simulink model "vectoring2023"  (R2023b)
settings: Solver=FixedStepAuto  StartTime=0.0  StopTime=10  FixedStep=0.001  RelTol=1e-3
undefined symbols (not defined in the file): DiscIntNeverNeededParam
libraries: simulink x4
(part 1 of 2)
settings Model: Creator=manda  LastModifiedBy=manda
settings DebuggingCC: AlgebraicLoopMsg=none  ArtificialAlgebraicLoopMsg=none
settings RTWCC: GPUComputeCapability=5.0

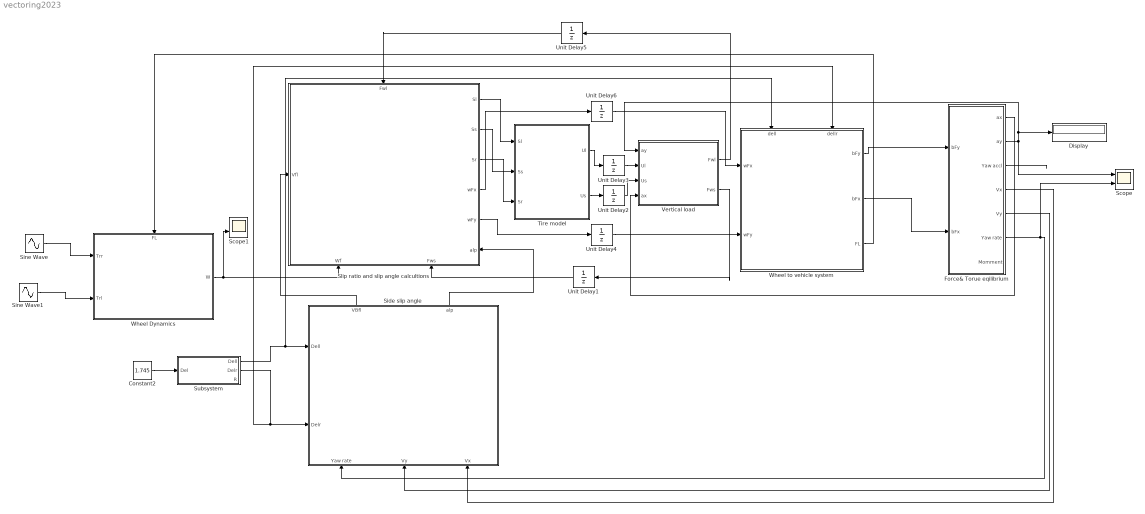
== system vectoring2023 ==
  Constant2 : Constant  Value=1.745
  Display : Display
  Force& Torue eqilibrium : Subsystem
  Scope : Scope  NumInputPorts=2
  Scope1 : Scope  NumInputPorts=2
  Side slip angle : Subsystem
      settings: PortSchema="{\"entries\":[{\"content\":{\"sides\":[{\"content\":{\"connectorIds\":[\"In1\",\"In2\",\"In3\"]},\"type\":\"ConnectorPlacement.EquallySpacedRectSide\",\"uuid\":\"ab28ffba-4240-48bb-9504-9e35b52ca467\"},{\"content\":{\"connectorIds\":[\"Out1\",\"Out2\"],\"side\":\"RIGHT\"},\"type\":\"ConnectorPlacement.EquallySpacedRectSide\",\"uuid\":\"e82fd81c-35f0-42c8-ade2-8771ec67db7c\"},{\"content\":{\"side\":\"TOP\"},\"type\":\"ConnectorPlacement.EquallySpacedRectSide\",\"uuid\":\"b58f2881-2655-4ae0-b45f-be5580c20129\"},{\"content\":{\"connectorIds\":[\"In4\",\"In5\"],\"side\":\"BOTTOM\"},\"type\":\"ConnectorPlacement.EquallySpacedRectSide\",\"uuid\":\"e7768be2-30e0-47b0-bc7d-0a1efc3645f2\"}]},\"type\":\"ConnectorPlacement.EquallySpacedConnector\",\"uuid\":\"813aa404-2cb1-4c8d-a503-6d07b8fe7df3\"}],\"packageUris\":[\"http://schema.mathworks.com/mf0/Connector/R2020b\"],\"version\":\"1.0\"}"
  Sine Wave : Sin  Amplitude=300  SampleTime=0
  Sine Wave1 : Sin  Amplitude=280  Frequency=2  SampleTime=0
  Slip ratio and slip angle calcultions : Subsystem
      settings: PortSchema="{\"entries\":[{\"content\":{\"sides\":[{\"content\":{\"connectorIds\":[\"In1\"]},\"type\":\"ConnectorPlacement.EquallySpacedRectSide\",\"uuid\":\"a7ec119f-fde6-41d0-ac79-405e8e24b01a\"},{\"content\":{\"connectorIds\":[\"Out1\",\"Out2\",\"Out3\",\"Out4\",\"Out5\",\"In5\"],\"side\":\"RIGHT\"},\"type\":\"ConnectorPlacement.EquallySpacedRectSide\",\"uuid\":\"f3b150d3-40b1-4a48-adf8-cf1c21578111\"},{\"content\":{\"connectorIds\":[\"In2\"],\"side\":\"TOP\"},\"type\":\"ConnectorPlacement.EquallySpacedRectSide\",\"uuid\":\"012c84a0-3b90-4200-9e2e-18642f8e7c8c\"},{\"content\":{\"connectorIds\":[\"In3\",\"In4\"],\"side\":\"BOTTOM\"},\"type\":\"ConnectorPlacement.EquallySpacedRectSide\",\"uuid\":\"07872eaa-713c-4fe8-8440-cce3cb3174e0\"}]},\"type\":\"ConnectorPlacement.EquallySpacedConnector\",\"uuid\":\"20f169d6-3b99-4690-9979-164201d75b1c\"}],\"packageUris\":[\"http://schema.mathworks.com/mf0/Connector/R2020b\"],\"version\":\"1.0\"}"
  Subsystem : Subsystem
  Tire model : Subsystem
  Unit Delay{1..6} (6 alike) : UnitDelay  SampleTime=-1  HasFrameUpgradeWarning=on
  "Vertical load " : Subsystem
  Wheel Dynamics : Subsystem
      settings: PortSchema="{\"entries\":[{\"content\":{\"sides\":[{\"content\":{\"connectorIds\":[\"In1\",\"In2\"]},\"type\":\"ConnectorPlacement.EquallySpacedRectSide\",\"uuid\":\"b5deda4c-2c89-449a-b9af-669b3c34e6b4\"},{\"content\":{\"connectorIds\":[\"Out1\"],\"side\":\"RIGHT\"},\"type\":\"ConnectorPlacement.EquallySpacedRectSide\",\"uuid\":\"37e39622-b3a7-494f-b6c8-82365593df34\"},{\"content\":{\"connectorIds\":[\"In3\"],\"side\":\"TOP\"},\"type\":\"ConnectorPlacement.EquallySpacedRectSide\",\"uuid\":\"023e6718-854f-4ad6-a520-bdc192d9d93c\"}]},\"type\":\"ConnectorPlacement.EquallySpacedConnector\",\"uuid\":\"2e43a3da-411d-4540-923d-79338234d95c\"}],\"packageUris\":[\"http://schema.mathworks.com/mf0/Connector/R2020b\"],\"version\":\"1.0\"}"
  Wheel to vehicle system : Subsystem
      settings: PortSchema="{\"entries\":[{\"content\":{\"sides\":[{\"content\":{\"connectorIds\":[\"In1\",\"In2\"]},\"type\":\"ConnectorPlacement.EquallySpacedRectSide\",\"uuid\":\"5c83ab18-6927-4337-9510-166b24334d1c\"},{\"content\":{\"connectorIds\":[\"Out1\",\"Out2\",\"Out3\"],\"side\":\"RIGHT\"},\"type\":\"ConnectorPlacement.EquallySpacedRectSide\",\"uuid\":\"a6e62921-01da-4957-9ce0-76b671842a08\"},{\"content\":{\"connectorIds\":[\"In3\",\"In4\"],\"side\":\"TOP\"},\"type\":\"ConnectorPlacement.EquallySpacedRectSide\",\"uuid\":\"6fd248c4-32bd-4a33-9140-17907c8186f8\"}]},\"type\":\"ConnectorPlacement.EquallySpacedConnector\",\"uuid\":\"96144e17-0eac-422a-892f-fd6e2a88ebc7\"}],\"packageUris\":[\"http://schema.mathworks.com/mf0/Connector/R2020b\"],\"version\":\"1.0\"}"
  wires:
  Slip ratio and slip angle calcultions/3(Sr) -> Tire model/3(Sr)
  "Vertical load "/1(Fwl) -> Unit Delay5/1
  Subsystem/1(Dell) -> Wheel to vehicle system/3(dell), Side slip angle/5(Dell)
  Subsystem/2(Delr) -> Side slip angle/4(Delr), Wheel to vehicle system/4(dellr)
  Constant2/1 -> Subsystem/1(Del)
  Force& Torue eqilibrium/6(Yaw rate) -> Scope/2, Side slip angle/3(Yaw rate)
  Force& Torue eqilibrium/1(ax) -> "Vertical load "/4(ax)
  Force& Torue eqilibrium/2(ay) -> "Vertical load "/1(ay), Display/1, Scope/1
  Side slip angle/1(alp) -> Slip ratio and slip angle calcultions/5(alp)
  Side slip angle/2(VBfl) -> Slip ratio and slip angle calcultions/1(Vfl)
  Slip ratio and slip angle calcultions/1(Sl) -> Tire model/1(Sl)
  Slip ratio and slip angle calcultions/2(Ss) -> Tire model/2(Ss)
  Force& Torue eqilibrium/4(Vx) -> Side slip angle/1(Vx)
  Force& Torue eqilibrium/5(Vy) -> Side slip angle/2(Vy)
  Sine Wave/1 -> Wheel Dynamics/1(Trr)
  Sine Wave1/1 -> Wheel Dynamics/2(Trl)
  Wheel Dynamics/1(W) -> Scope1/2, Slip ratio and slip angle calcultions/3(Wf)
  Tire model/2(Us) -> Unit Delay2/1
  Unit Delay2/1 -> "Vertical load "/3(Us)
  Tire model/1(Ul) -> Unit Delay3/1
  Unit Delay3/1 -> "Vertical load "/2(Ul)
  Unit Delay5/1 -> Slip ratio and slip angle calcultions/2(Fwl)
  Slip ratio and slip angle calcultions/5(wFy) -> Unit Delay4/1
  Slip ratio and slip angle calcultions/4(wFx) -> Unit Delay6/1
  "Vertical load "/2(Fws) -> Unit Delay1/1
  Unit Delay1/1 -> Slip ratio and slip angle calcultions/4(Fws)
  Unit Delay4/1 -> Wheel to vehicle system/2(wFy)
  Unit Delay6/1 -> Wheel to vehicle system/1(wFx)
  Wheel to vehicle system/1(bFy) -> Force& Torue eqilibrium/1(bFy)
  Wheel to vehicle system/2(bFx) -> Force& Torue eqilibrium/2(bFx)
  Force& Torue eqilibrium/3(Yaw accl) -> ?
  Wheel to vehicle system/3(FL) -> Wheel Dynamics/3(FL)

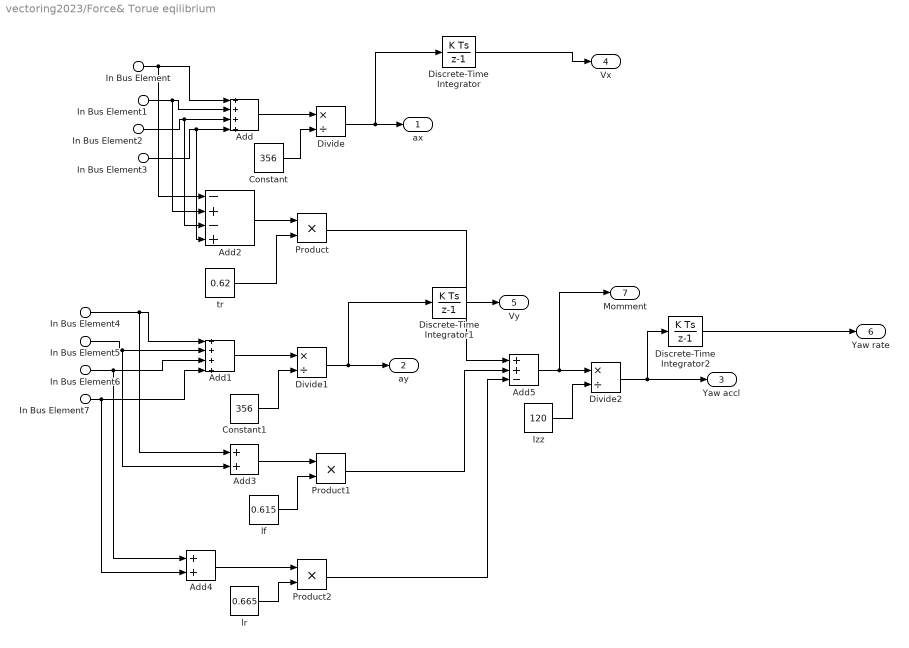
== system vectoring2023/Force& Torue eqilibrium ==
  In Bus Element4 : Inport  PortName=bFy  Element=bFy;fl
  In Bus Element5 : Inport  PortName=bFy  Element=bFy;fr
  In Bus Element6 : Inport  PortName=bFy  Element=Fwy;rl
  In Bus Element7 : Inport  PortName=bFy  Element=Fwy;rr
  In Bus Element : Inport  Port=2  PortName=bFx  Element=bFx;fl
  In Bus Element1 : Inport  Port=2  PortName=bFx  Element=bFx;fr
  In Bus Element2 : Inport  Port=2  PortName=bFx  Element=Fwx;rl
  In Bus Element3 : Inport  Port=2  PortName=bFx  Element=Fwx;rr
  Add : Sum  Inputs=++++
  Add1 : Sum  Inputs=++++
  Add2 : Sum  Inputs=-+-+
  Add3 : Sum
  Add4 : Sum
  Add5 : Sum  Inputs=++-
  Constant : Constant  Value=356
  Constant1 : Constant  Value=356
  Discrete-Time Integrator : DiscreteIntegrator  SampleTime=-1  ICPrevOutput=DiscIntNeverNeededParam  ICPrevScaledInput=DiscIntNeverNeededParam
  Discrete-Time Integrator1 : DiscreteIntegrator  SampleTime=-1  ICPrevOutput=DiscIntNeverNeededParam  ICPrevScaledInput=DiscIntNeverNeededParam
  Discrete-Time Integrator2 : DiscreteIntegrator  SampleTime=-1  ICPrevOutput=DiscIntNeverNeededParam  ICPrevScaledInput=DiscIntNeverNeededParam
  Divide : Product  Inputs=*/
  Divide1 : Product  Inputs=*/
  Divide2 : Product  Inputs=*/
  Izz : Constant  Value=120
  Product : Product
  Product1 : Product
  Product2 : Product
  lf : Constant  Value=0.615
  lr : Constant  Value=0.665
  tr : Constant  Value=0.62
  ax : Outport
  ay : Outport  Port=2
  Yaw accl : Outport  Port=3
  Vx : Outport  Port=4
  Vy : Outport  Port=5
  Yaw rate : Outport  Port=6
  Momment : Outport  Port=7
  wires:
  In Bus Element2/1 -> Add2/3, Add/3
  In Bus Element/1 -> Add2/1, Add/1
  In Bus Element1/1 -> Add2/2, Add/2
  In Bus Element3/1 -> Add2/4, Add/4
  Add/1 -> Divide/1
  Constant/1 -> Divide/2
  Divide/1 -> Discrete-Time Integrator/1, ax/1
  In Bus Element4/1 -> Add3/1, Add1/1
  In Bus Element6/1 -> Add4/1, Add1/3
  In Bus Element7/1 -> Add4/2, Add1/4
  Add1/1 -> Divide1/1
  Constant1/1 -> Divide1/2
  Add2/1 -> Product/1
  tr/1 -> Product/2
  In Bus Element5/1 -> Add3/2, Add1/2
  Add3/1 -> Product1/1
  lf/1 -> Product1/2
  Add4/1 -> Product2/1
  lr/1 -> Product2/2
  Product/1 -> Add5/1
  Product1/1 -> Add5/2
  Product2/1 -> Add5/3
  Add5/1 -> Momment/1, Divide2/1
  Izz/1 -> Divide2/2
  Divide2/1 -> Discrete-Time Integrator2/1, Yaw accl/1
  Discrete-Time Integrator/1 -> Vx/1
  Discrete-Time Integrator1/1 -> Vy/1
  Discrete-Time Integrator2/1 -> Yaw rate/1
  Divide1/1 -> Discrete-Time Integrator1/1, ay/1

== system vectoring2023/Side slip angle ==
  Vx : Inport
  Vy : Inport  Port=2
  Yaw rate : Inport  Port=3
  Delr : Inport  Port=4
  Dell : Inport  Port=5
  Radius of wheel point from center : Subsystem
  Vel of whee due to veh speedl : Subsystem
  alpfl Subsystem : Subsystem
  alpfr Subsystem : Subsystem
  alprl Subsystem : Subsystem
  alprr Subsystem1 : Subsystem
  Out Bus Element : Outport  PortName=alp  Element=alpfl
  Out Bus Element1 : Outport  PortName=alp  Element=alprr
  Out Bus Element2 : Outport  PortName=alp  Element=alprl
  Out Bus Element3 : Outport  PortName=alp  Element=alpfr
  Out Bus Element4 : Outport  Port=2  PortName=VBfl  Element=VBfl
  Out Bus Element5 : Outport  Port=2  PortName=VBfl  Element=VBfr
  Out Bus Element6 : Outport  Port=2  PortName=VBfl  Element=VBrl
  Out Bus Element7 : Outport  Port=2  PortName=VBfl  Element=VBrr
  wires:
  Radius of wheel point from center/1(Rfcenter) -> alpfr Subsystem/1(Rfcenter), alpfl Subsystem/1(Rfc), alpfr Subsystem/2(In2), alpfl Subsystem/2(In2), Vel of whee due to veh speedl/8(Rfcenter)
  Radius of wheel point from center/2(Rrc) -> alprr Subsystem1/2(In2), alprr Subsystem1/1(Rrc), alprl Subsystem/2(In2), Vel of whee due to veh speedl/7(Rrc), alprl Subsystem/1(Rrc)
  Radius of wheel point from center/3(efl) -> Vel of whee due to veh speedl/2(efl), alpfl Subsystem/3(efl)
  Vx/1 -> Vel of whee due to veh speedl/9(Vx), alprl Subsystem/4(Vx), alprr Subsystem1/4(Vx), alpfr Subsystem/4(Vx), alpfl Subsystem/4(Vx)
  Vy/1 -> Vel of whee due to veh speedl/1(Vy), alprr Subsystem1/5(Vy), alpfr Subsystem/5(Vy), alpfl Subsystem/5(Vy), alprl Subsystem/5(Vy)
  alpfl Subsystem/1(alpfl) -> Out Bus Element/1
  Dell/1 -> alpfl Subsystem/7(Dell)
  Delr/1 -> alpfr Subsystem/7(Delr)
  Radius of wheel point from center/4(efr) -> Vel of whee due to veh speedl/3(efr), alpfr Subsystem/3(efr)
  alpfr Subsystem/1(alpfr) -> Out Bus Element3/1
  Radius of wheel point from center/5(erl) -> alprl Subsystem/3(erl), Vel of whee due to veh speedl/5(erl)
  Radius of wheel point from center/6(err) -> alprr Subsystem1/3(err), Vel of whee due to veh speedl/4(err)
  alprl Subsystem/1(alprl) -> Out Bus Element2/1
  alprr Subsystem1/1(alprr) -> Out Bus Element1/1
  Yaw rate/1 -> Vel of whee due to veh speedl/6(Yaw rate), alpfr Subsystem/6(Yaw rate), alpfl Subsystem/6(Yaw rate), alprr Subsystem1/6(Yaw rate), alprl Subsystem/6(Yaw rate)
  Vel of whee due to veh speedl/1(VBfl) -> Out Bus Element4/1
  Vel of whee due to veh speedl/2(VBfr) -> Out Bus Element5/1
  Vel of whee due to veh speedl/3(VBrl) -> Out Bus Element6/1
  Vel of whee due to veh speedl/4(VBrr) -> Out Bus Element7/1

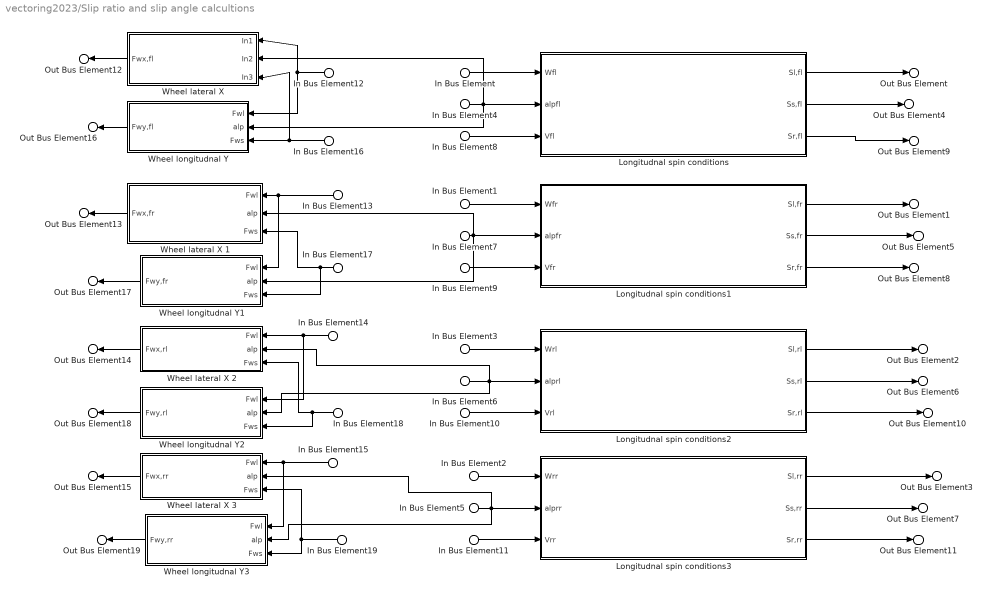
== system vectoring2023/Slip ratio and slip angle calcultions ==
  In Bus Element8 : Inport  PortName=Vfl  Element=VBfl
  In Bus Element9 : Inport  PortName=Vfl  Element=VBfr
  In Bus Element10 : Inport  PortName=Vfl  Element=VBrl
  In Bus Element11 : Inport  PortName=Vfl  Element=VBrr
  In Bus Element12 : Inport  Port=2  PortName=Fwl  Element=Fwl;fl
  In Bus Element13 : Inport  Port=2  PortName=Fwl  Element=Fwl;fr
  In Bus Element14 : Inport  Port=2  PortName=Fwl  Element=Fwl;rl
  In Bus Element15 : Inport  Port=2  PortName=Fwl  Element=Fwl;rr
  In Bus Element : Inport  Port=3  PortName=Wf  Element=Wfl
  In Bus Element1 : Inport  Port=3  PortName=Wf  Element=Wfr
  In Bus Element2 : Inport  Port=3  PortName=Wf  Element=Wrr
  In Bus Element3 : Inport  Port=3  PortName=Wf  Element=Wrl
  In Bus Element16 : Inport  Port=4  PortName=Fws  Element=Fws;fl
  In Bus Element17 : Inport  Port=4  PortName=Fws  Element=Fws;fr
  In Bus Element18 : Inport  Port=4  PortName=Fws  Element=Fws;rl
  In Bus Element19 : Inport  Port=4  PortName=Fws  Element=Fwl;rr
  In Bus Element4 : Inport  Port=5  PortName=alp  Element=alpfl
  In Bus Element5 : Inport  Port=5  PortName=alp  Element=alprr
  In Bus Element6 : Inport  Port=5  PortName=alp  Element=alprl
  In Bus Element7 : Inport  Port=5  PortName=alp  Element=alpfr
  Longitudnal spin conditions : Subsystem
  Longitudnal spin conditions1 : Subsystem
  Longitudnal spin conditions2 : Subsystem
  Longitudnal spin conditions3 : Subsystem
  "Wheel lateral X " : Subsystem
  Wheel lateral X 1 : Subsystem
  Wheel lateral X 2 : Subsystem
  Wheel lateral X 3 : Subsystem
  Wheel longitudnal Y : Subsystem
  Wheel longitudnal Y1 : Subsystem
  Wheel longitudnal Y2 : Subsystem
  Wheel longitudnal Y3 : Subsystem
  Out Bus Element : Outport  PortName=Sl  Element=Sl;fl
  Out Bus Element1 : Outport  PortName=Sl  Element=Sl;fr
  Out Bus Element2 : Outport  PortName=Sl  Element=Sl;rl
  Out Bus Element3 : Outport  PortName=Sl  Element=Sl;rr
  Out Bus Element4 : Outport  Port=2  PortName=Ss  Element=Ss;fl
  Out Bus Element5 : Outport  Port=2  PortName=Ss  Element=Ss;fr
  Out Bus Element6 : Outport  Port=2  PortName=Ss  Element=Ss;rl
  Out Bus Element7 : Outport  Port=2  PortName=Ss  Element=Ss;rr
  Out Bus Element8 : Outport  Port=3  PortName=Sr  Element=Sr;fr
  Out Bus Element9 : Outport  Port=3  PortName=Sr  Element=Sr;fl
  Out Bus Element10 : Outport  Port=3  PortName=Sr  Element=Sr;rl
  Out Bus Element11 : Outport  Port=3  PortName=Sr  Element=Sr;rr
  Out Bus Element12 : Outport  Port=4  PortName=wFx  Element=Fwx;fl
  Out Bus Element13 : Outport  Port=4  PortName=wFx  Element=Fwx;fr
  Out Bus Element14 : Outport  Port=4  PortName=wFx  Element=Fwx;rl
  Out Bus Element15 : Outport  Port=4  PortName=wFx  Element=Fwx;rr
  Out Bus Element16 : Outport  Port=5  PortName=wFy  Element=Fwy;fl
  Out Bus Element17 : Outport  Port=5  PortName=wFy  Element=Fwy;fr
  Out Bus Element18 : Outport  Port=5  PortName=wFy  Element=Fwy;rl
  Out Bus Element19 : Outport  Port=5  PortName=wFy  Element=Fwy;rr
  wires:
  In Bus Element/1 -> Longitudnal spin conditions/1(Wfl)
  In Bus Element4/1 -> Wheel longitudnal Y/2(alp), "Wheel lateral X "/2(In2), Longitudnal spin conditions/2(alpfl)
  In Bus Element8/1 -> Longitudnal spin conditions/3(Vfl)
  In Bus Element1/1 -> Longitudnal spin conditions1/1(Wfr)
  In Bus Element7/1 -> Wheel longitudnal Y1/2(alp), Longitudnal spin conditions1/2(alpfr), Wheel lateral X 1/2(alp)
  In Bus Element9/1 -> Longitudnal spin conditions1/3(Vfr)
  In Bus Element10/1 -> Longitudnal spin conditions2/3(Vrl)
  In Bus Element6/1 -> Wheel longitudnal Y2/2(alp), Wheel lateral X 2/2(alp), Longitudnal spin conditions2/2(alprl)
  In Bus Element3/1 -> Longitudnal spin conditions2/1(Wrl)
  In Bus Element2/1 -> Longitudnal spin conditions3/1(Wrr)
  In Bus Element11/1 -> Longitudnal spin conditions3/3(Vrr)
  Longitudnal spin conditions/1(Sl,fl) -> Out Bus Element/1
  Longitudnal spin conditions1/1(Sl,fr) -> Out Bus Element1/1
  Longitudnal spin conditions2/1(Sl,rl) -> Out Bus Element2/1
  Longitudnal spin conditions3/1(Sl,rr) -> Out Bus Element3/1
  Longitudnal spin conditions/2(Ss,fl) -> Out Bus Element4/1
  Longitudnal spin conditions1/2(Ss,fr) -> Out Bus Element5/1
  Longitudnal spin conditions2/2(Ss,rl) -> Out Bus Element6/1
  Longitudnal spin conditions3/2(Ss,rr) -> Out Bus Element7/1
  Longitudnal spin conditions/3(Sr,fl) -> Out Bus Element9/1
  Longitudnal spin conditions1/3(Sr,fr) -> Out Bus Element8/1
  Longitudnal spin conditions2/3(Sr,rl) -> Out Bus Element10/1
  Longitudnal spin conditions3/3(Sr,rr) -> Out Bus Element11/1
  In Bus Element5/1 -> Wheel longitudnal Y3/2(alp), Wheel lateral X 3/2(alp), Longitudnal spin conditions3/2(alprr)
  In Bus Element12/1 -> "Wheel lateral X "/1(In1), Wheel longitudnal Y/1(Fwl)
  In Bus Element16/1 -> Wheel longitudnal Y/3(Fws), "Wheel lateral X "/3(In3)
  "Wheel lateral X "/1(Fwx,fl) -> Out Bus Element12/1
  In Bus Element13/1 -> Wheel longitudnal Y1/1(Fwl), Wheel lateral X 1/1(Fwl)
  In Bus Element17/1 -> Wheel longitudnal Y1/3(Fws), Wheel lateral X 1/3(Fws)
  Wheel lateral X 1/1(Fwx,fr) -> Out Bus Element13/1
  In Bus Element14/1 -> Wheel longitudnal Y2/1(Fwl), Wheel lateral X 2/1(Fwl)
  In Bus Element18/1 -> Wheel longitudnal Y2/3(Fws), Wheel lateral X 2/3(Fws)
  Wheel lateral X 2/1(Fwx,rl) -> Out Bus Element14/1
  In Bus Element15/1 -> Wheel longitudnal Y3/1(Fwl), Wheel lateral X 3/1(Fwl)
  In Bus Element19/1 -> Wheel longitudnal Y3/3(Fws), Wheel lateral X 3/3(Fws)
  Wheel lateral X 3/1(Fwx,rr) -> Out Bus Element15/1
  Wheel longitudnal Y/1(Fwy,fl) -> Out Bus Element16/1
  Wheel longitudnal Y1/1(Fwy,fr) -> Out Bus Element17/1
  Wheel longitudnal Y2/1(Fwy,rl) -> Out Bus Element18/1
  Wheel longitudnal Y3/1(Fwy,rr) -> Out Bus Element19/1

== system vectoring2023/Subsystem ==
  Del : Inport
  Divide : Product  Inputs=*/
  Divide1 : Product  Inputs=*/
  Divide2 : Product  Inputs=*/
  Math Function : Math  Operator=square
  Math Function1 : Math  Operator=square
  Sqrt : Sqrt
  Subtract : Sum  Inputs=+-
  Subtract1 : Sum
  Subtract2 : Sum
  Trigonometric Function : Trigonometry  Operator=tan
  l : Constant  Value=1.29
  tf/2 : Constant  Value=0.31
  Dell : Outport
  Delr : Outport  Port=2
  R : Outport  Port=3
  wires:
  Del/1 -> Trigonometric Function/1
  l/1 -> Divide2/1, Divide/1, Divide1/1
  Trigonometric Function/1 -> Divide1/2
  Divide1/1 -> Math Function/1, Subtract1/1, Subtract/1
  tf/2/1 -> Subtract/2, Math Function1/1, Subtract1/2
  Subtract/1 -> Divide/2
  Divide/1 -> Dell/1
  Subtract1/1 -> Divide2/2
  Divide2/1 -> Delr/1
  Math Function/1 -> Subtract2/1
  Math Function1/1 -> Subtract2/2
  Sqrt/1 -> R/1
  Subtract2/1 -> Sqrt/1

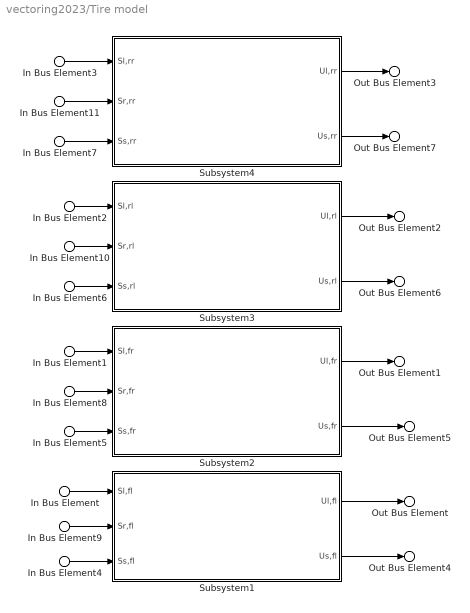
== system vectoring2023/Tire model ==
  In Bus Element : Inport  PortName=Sl  Element=Sl;fl
  In Bus Element1 : Inport  PortName=Sl  Element=Sl;fr
  In Bus Element2 : Inport  PortName=Sl  Element=Sl;rl
  In Bus Element3 : Inport  PortName=Sl  Element=Sl;rr
  In Bus Element4 : Inport  Port=2  PortName=Ss  Element=Ss;fl
  In Bus Element5 : Inport  Port=2  PortName=Ss  Element=Ss;fr
  In Bus Element6 : Inport  Port=2  PortName=Ss  Element=Ss;rl
  In Bus Element7 : Inport  Port=2  PortName=Ss  Element=Ss;rr
  In Bus Element8 : Inport  Port=3  PortName=Sr  Element=Sr;fr
  In Bus Element9 : Inport  Port=3  PortName=Sr  Element=Sr;fl
  In Bus Element10 : Inport  Port=3  PortName=Sr  Element=Sr;rl
  In Bus Element11 : Inport  Port=3  PortName=Sr  Element=Sr;rr
  Subsystem1 : Subsystem
  Subsystem2 : Subsystem
  Subsystem3 : Subsystem
  Subsystem4 : Subsystem
  Out Bus Element : Outport  PortName=Ul  Element=Ul;fl
  Out Bus Element1 : Outport  PortName=Ul  Element=Ul;fr
  Out Bus Element2 : Outport  PortName=Ul  Element=Ul;rl
  Out Bus Element3 : Outport  PortName=Ul  Element=Ul;rr
  Out Bus Element4 : Outport  Port=2  PortName=Us  Element=Us;fl
  Out Bus Element5 : Outport  Port=2  PortName=Us  Element=Us;fr
  Out Bus Element6 : Outport  Port=2  PortName=Us  Element=Us;rl
  Out Bus Element7 : Outport  Port=2  PortName=Us  Element=Us;rr
  wires:
  In Bus Element1/1 -> Subsystem2/1(Sl,fr)
  In Bus Element/1 -> Subsystem1/1(Sl,fl)
  In Bus Element9/1 -> Subsystem1/2(Sr,fl)
  In Bus Element4/1 -> Subsystem1/3(Ss,fl)
  Subsystem1/2(Us,fl) -> Out Bus Element4/1
  In Bus Element8/1 -> Subsystem2/2(Sr,fr)
  In Bus Element5/1 -> Subsystem2/3(Ss,fr)
  In Bus Element2/1 -> Subsystem3/1(Sl,rl)
  In Bus Element10/1 -> Subsystem3/2(Sr,rl)
  In Bus Element6/1 -> Subsystem3/3(Ss,rl)
  In Bus Element11/1 -> Subsystem4/2(Sr,rr)
  In Bus Element7/1 -> Subsystem4/3(Ss,rr)
  In Bus Element3/1 -> Subsystem4/1(Sl,rr)
  Subsystem2/2(Us,fr) -> Out Bus Element5/1
  Subsystem3/2(Us,rl) -> Out Bus Element6/1
  Subsystem4/2(Us,rr) -> Out Bus Element7/1
  Subsystem1/1(Ul,fl) -> Out Bus Element/1
  Subsystem2/1(Ul,fr) -> Out Bus Element1/1
  Subsystem3/1(Ul,rl) -> Out Bus Element2/1
  Subsystem4/1(Ul,rr) -> Out Bus Element3/1

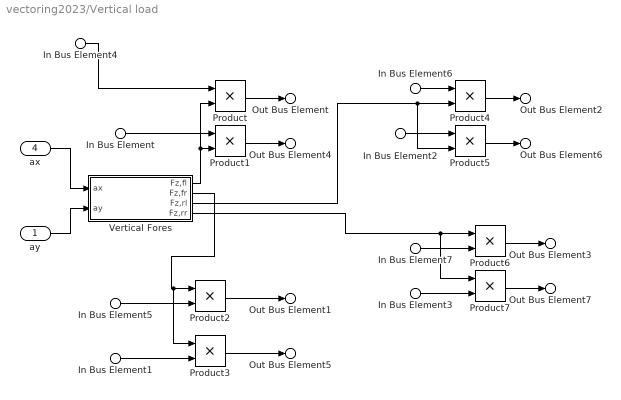
== system vectoring2023/Vertical load  ==
  ay : Inport
  In Bus Element4 : Inport  Port=2  PortName=Ul  Element=Ul;fl
  In Bus Element5 : Inport  Port=2  PortName=Ul  Element=Ul;fr
  In Bus Element6 : Inport  Port=2  PortName=Ul  Element=Ul;rl
  In Bus Element7 : Inport  Port=2  PortName=Ul  Element=Ul;rr
  In Bus Element : Inport  Port=3  PortName=Us  Element=Us;fl
  In Bus Element1 : Inport  Port=3  PortName=Us  Element=Us;fr
  In Bus Element2 : Inport  Port=3  PortName=Us  Element=Us;rl
  In Bus Element3 : Inport  Port=3  PortName=Us  Element=Us;rr
  ax : Inport  Port=4
  Product{,1..7} (8 alike) : Product
  Vertical Fores : Subsystem
  Out Bus Element : Outport  PortName=Fwl  Element=Fwl;fl
  Out Bus Element1 : Outport  PortName=Fwl  Element=Fwl;fr
  Out Bus Element2 : Outport  PortName=Fwl  Element=Fwl;rl
  Out Bus Element3 : Outport  PortName=Fwl  Element=Fwl;rr
  Out Bus Element4 : Outport  Port=2  PortName=Fws  Element=Fws;fl
  Out Bus Element5 : Outport  Port=2  PortName=Fws  Element=Fws;fr
  Out Bus Element6 : Outport  Port=2  PortName=Fws  Element=Fws;rl
  Out Bus Element7 : Outport  Port=2  PortName=Fws  Element=Fwl;rr
  wires:
  ay/1 -> Vertical Fores/2(ay)
  ax/1 -> Vertical Fores/1(ax)
  In Bus Element4/1 -> Product/1
  Vertical Fores/1(Fz,fl) -> Product/2, Product1/2
  Product/1 -> Out Bus Element/1
  In Bus Element/1 -> Product1/1
  Product1/1 -> Out Bus Element4/1
  In Bus Element5/1 -> Product2/2
  Vertical Fores/2(Fz,fr) -> Product3/1, Product2/1
  Product2/1 -> Out Bus Element1/1
  In Bus Element1/1 -> Product3/2
  Product3/1 -> Out Bus Element5/1
  In Bus Element6/1 -> Product4/1
  Vertical Fores/3(Fz,rl) -> Product5/2, Product4/2
  Product4/1 -> Out Bus Element2/1
  In Bus Element2/1 -> Product5/1
  Product5/1 -> Out Bus Element6/1
  In Bus Element7/1 -> Product6/2
  Vertical Fores/4(Fz,rr) -> Product7/1, Product6/1
  Product6/1 -> Out Bus Element3/1
  In Bus Element3/1 -> Product7/2
  Product7/1 -> Out Bus Element7/1

== system vectoring2023/Wheel Dynamics ==
  Trr : Inport
  Trl : Inport  Port=2
  In Bus Element : Inport  Port=3  PortName=FL  Element=fl
  In Bus Element1 : Inport  Port=3  PortName=FL  Element=rl
  In Bus Element2 : Inport  Port=3  PortName=FL  Element=fr
  In Bus Element3 : Inport  Port=3  PortName=FL  Element=rr
  Wfl subsystem : Subsystem
  Wfr subsytem : Subsystem
  Wrl subsystem : Subsystem
  Wrr Subsystem : Subsystem
  Out Bus Element : Outport  PortName=W  Element=Wfl
  Out Bus Element1 : Outport  PortName=W  Element=Wfr
  Out Bus Element2 : Outport  PortName=W  Element=Wrr
  Out Bus Element3 : Outport  PortName=W  Element=Wrl
  wires:
  In Bus Element/1 -> Wfl subsystem/1(Ffl)
  Wfl subsystem/1(Wfl) -> Out Bus Element/1
  In Bus Element2/1 -> Wfr subsytem/1(Ffr)
  Trl/1 -> Wrl subsystem/1(Trl)
  In Bus Element1/1 -> Wrl subsystem/2(Frl)
  Wrl subsystem/1(Wrl) -> Out Bus Element3/1
  Trr/1 -> Wrr Subsystem/1(Trr)
  In Bus Element3/1 -> Wrr Subsystem/2(Frr)
  Wrr Subsystem/1(Wrr) -> Out Bus Element2/1
  Wfr subsytem/1(Wfr) -> Out Bus Element1/1

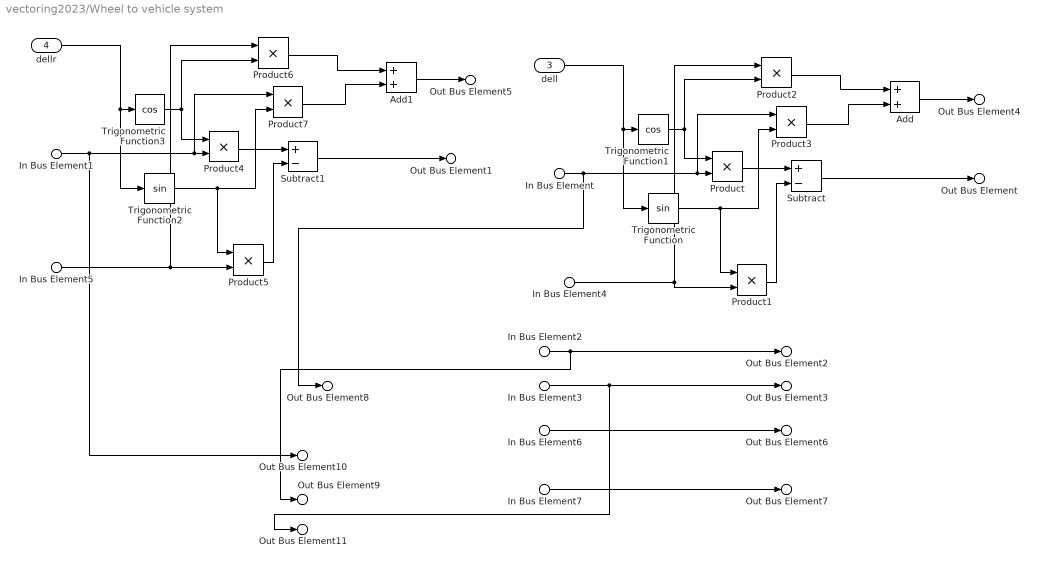
== system vectoring2023/Wheel to vehicle system ==
  In Bus Element : Inport  PortName=wFx  Element=Fwx;fl
  In Bus Element1 : Inport  PortName=wFx  Element=Fwx;fr
  In Bus Element2 : Inport  PortName=wFx  Element=Fwx;rl
  In Bus Element3 : Inport  PortName=wFx  Element=Fwx;rr
  In Bus Element4 : Inport  Port=2  PortName=wFy  Element=Fwy;fl
  In Bus Element5 : Inport  Port=2  PortName=wFy  Element=Fwy;fr
  In Bus Element6 : Inport  Port=2  PortName=wFy  Element=Fwy;rl
  In Bus Element7 : Inport  Port=2  PortName=wFy  Element=Fwy;rr
  dell : Inport  Port=3
  dellr : Inport  Port=4
  Add : Sum
  Add1 : Sum
  Product{,1..7} (8 alike) : Product
  Subtract : Sum  Inputs=+-
  Subtract1 : Sum  Inputs=+-
  Trigonometric Function : Trigonometry
  Trigonometric Function1 : Trigonometry  Operator=cos
  Trigonometric Function2 : Trigonometry
  Trigonometric Function3 : Trigonometry  Operator=cos
  Out Bus Element4 : Outport  PortName=bFy  Element=bFy;fl
  Out Bus Element5 : Outport  PortName=bFy  Element=bFy;fr
  Out Bus Element6 : Outport  PortName=bFy  Element=Fwy;rl
  Out Bus Element7 : Outport  PortName=bFy  Element=Fwy;rr
  Out Bus Element : Outport  Port=2  PortName=bFx  Element=bFx;fl
  Out Bus Element1 : Outport  Port=2  PortName=bFx  Element=bFx;fr
  Out Bus Element2 : Outport  Port=2  PortName=bFx  Element=Fwx;rl
  Out Bus Element3 : Outport  Port=2  PortName=bFx  Element=Fwx;rr
  Out Bus Element8 : Outport  Port=3  PortName=FL  Element=fl
  Out Bus Element9 : Outport  Port=3  PortName=FL  Element=rl
  Out Bus Element10 : Outport  Port=3  PortName=FL  Element=fr
  Out Bus Element11 : Outport  Port=3  PortName=FL  Element=rr
  wires:
  dell/1 -> Trigonometric Function/1, Trigonometric Function1/1
  Trigonometric Function1/1 -> Product/1, Product2/2
  In Bus Element/1 -> Out Bus Element8/1, Product3/1, Product/2
  Product/1 -> Subtract/1
  Trigonometric Function/1 -> Product1/1, Product3/2
  In Bus Element4/1 -> Product1/2, Product2/1
  Product1/1 -> Subtract/2
  Subtract/1 -> Out Bus Element/1
  In Bus Element7/1 -> Out Bus Element7/1
  In Bus Element6/1 -> Out Bus Element6/1
  In Bus Element3/1 -> Out Bus Element11/1, Out Bus Element3/1
  In Bus Element2/1 -> Out Bus Element9/1, Out Bus Element2/1
  Product3/1 -> Add/2
  Product2/1 -> Add/1
  Add/1 -> Out Bus Element4/1
  Add1/1 -> Out Bus Element5/1
  Product6/1 -> Add1/1
  Product7/1 -> Add1/2
  Subtract1/1 -> Out Bus Element1/1
  Product5/1 -> Subtract1/2
  In Bus Element5/1 -> Product6/1, Product5/2
  Trigonometric Function2/1 -> Product7/2, Product5/1
  Product4/1 -> Subtract1/1
  In Bus Element1/1 -> Out Bus Element10/1, Product4/2, Product7/1
  Trigonometric Function3/1 -> Product6/2, Product4/1
  dellr/1 -> Trigonometric Function3/1, Trigonometric Function2/1

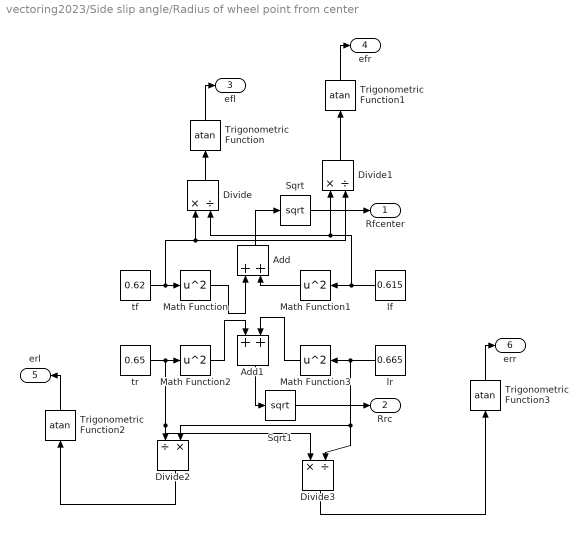
== system vectoring2023/Side slip angle/Radius of wheel point from center ==
  Add : Sum
  Add1 : Sum
  Divide{,1..3} (4 alike) : Product  Inputs=*/
  Math Function{,1..3} (4 alike) : Math  Operator=square
  Sqrt : Sqrt
  Sqrt1 : Sqrt
  Trigonometric Function{,1..3} (4 alike) : Trigonometry  Operator=atan
  lf : Constant  Value=0.615
  lr : Constant  Value=0.665
  tf : Constant  Value=0.62
  tr : Constant  Value=0.65
  Rfcenter : Outport
  Rrc : Outport  Port=2
  efl : Outport  Port=3
  efr : Outport  Port=4
  erl : Outport  Port=5
  err : Outport  Port=6
  wires:
  Sqrt/1 -> Rfcenter/1
  Math Function/1 -> Add/1
  Math Function2/1 -> Add1/1
  lf/1 -> Divide1/1, Divide/2, Math Function1/1
  tr/1 -> Divide3/1, Divide2/2, Math Function2/1
  lr/1 -> Divide3/2, Divide2/1, Math Function3/1
  Add1/1 -> Sqrt1/1
  tf/1 -> Divide1/2, Divide/1, Math Function/1
  Math Function3/1 -> Add1/2
  Add/1 -> Sqrt/1
  Sqrt1/1 -> Rrc/1
  Math Function1/1 -> Add/2
  Divide/1 -> Trigonometric Function/1
  Trigonometric Function/1 -> efl/1
  Trigonometric Function1/1 -> efr/1
  Divide1/1 -> Trigonometric Function1/1
  Trigonometric Function2/1 -> erl/1
  Divide2/1 -> Trigonometric Function2/1
  Trigonometric Function3/1 -> err/1
  Divide3/1 -> Trigonometric Function3/1

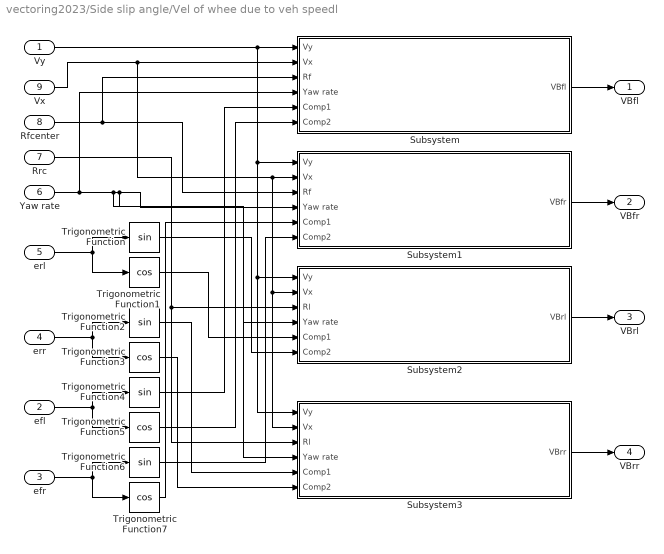
== system vectoring2023/Side slip angle/Vel of whee due to veh speedl ==
  Vy : Inport
  efl : Inport  Port=2
  efr : Inport  Port=3
  err : Inport  Port=4
  erl : Inport  Port=5
  Yaw rate : Inport  Port=6
  Rrc : Inport  Port=7
  Rfcenter : Inport  Port=8
  Vx : Inport  Port=9
  Subsystem : Subsystem
  Subsystem1 : Subsystem
  Subsystem2 : Subsystem
  Subsystem3 : Subsystem
  Trigonometric Function{,2,4,6} (4 alike) : Trigonometry
  Trigonometric Function{1,3,5,7} (4 alike) : Trigonometry  Operator=cos
  VBfl : Outport
  VBfr : Outport  Port=2
  VBrl : Outport  Port=3
  VBrr : Outport  Port=4
  wires:
  erl/1 -> Trigonometric Function/1, Trigonometric Function1/1
  err/1 -> Trigonometric Function2/1, Trigonometric Function3/1
  efl/1 -> Trigonometric Function5/1, Trigonometric Function4/1
  efr/1 -> Trigonometric Function6/1, Trigonometric Function7/1
  Vy/1 -> Subsystem3/1(Vy), Subsystem2/1(Vy), Subsystem1/1(Vy), Subsystem/1(Vy)
  Vx/1 -> Subsystem3/2(Vx), Subsystem2/2(Vx), Subsystem1/2(Vx), Subsystem/2(Vx)
  Rfcenter/1 -> Subsystem1/3(Rf), Subsystem/3(Rf)
  Trigonometric Function4/1 -> Subsystem/5(Comp1)
  Trigonometric Function5/1 -> Subsystem/6(Comp2)
  Subsystem/1(VBfl) -> VBfl/1
  Trigonometric Function7/1 -> Subsystem1/5(Comp1)
  Trigonometric Function6/1 -> Subsystem1/6(Comp2)
  Subsystem1/1(VBfr) -> VBfr/1
  Rrc/1 -> Subsystem3/3(Rl), Subsystem2/3(Rl)
  Yaw rate/1 -> Subsystem2/4(Yaw rate), Subsystem1/4(Yaw rate), Subsystem3/4(Yaw rate), Subsystem/4(Yaw rate)
  Trigonometric Function1/1 -> Subsystem2/5(Comp1)
  Trigonometric Function/1 -> Subsystem2/6(Comp2)
  Subsystem2/1(VBrl) -> VBrl/1
  Subsystem3/1(VBrr) -> VBrr/1
  Trigonometric Function2/1 -> Subsystem3/5(Comp1)
  Trigonometric Function3/1 -> Subsystem3/6(Comp2)

== system vectoring2023/Side slip angle/alpfl Subsystem ==
  Rfc : Inport
  In2 : Inport  Port=2
  efl : Inport  Port=3
  Vx : Inport  Port=4
  Vy : Inport  Port=5
  Yaw rate : Inport  Port=6
  Dell : Inport  Port=7
  Add : Sum
  Add1 : Sum  Inputs=+-
  Add2 : Sum  Inputs=+-
  Divide : Product  Inputs=*/
  Product : Product  Inputs=3
  Product1 : Product  Inputs=3
  Trigonometric Function : Trigonometry  Operator=cos
  Trigonometric Function1 : Trigonometry
  Trigonometric Function2 : Trigonometry  Operator=atan
  alpfl : Outport
  wires:
  Yaw rate/1 -> Product1/1, Product/1
  Vy/1 -> Add/1
  efl/1 -> Trigonometric Function1/1, Trigonometric Function/1
  Vx/1 -> Add1/1
  Product/1 -> Add/2
  Rfc/1 -> Product1/2
  Trigonometric Function1/1 -> Product1/3
  Add/1 -> Divide/1
  Product1/1 -> Add1/2
  Divide/1 -> Trigonometric Function2/1
  Trigonometric Function/1 -> Product/3
  Add1/1 -> Divide/2
  In2/1 -> Product/2
  Trigonometric Function2/1 -> Add2/2
  Dell/1 -> Add2/1
  Add2/1 -> alpfl/1

== system vectoring2023/Side slip angle/alpfr Subsystem ==
  Rfcenter : Inport
  In2 : Inport  Port=2
  efr : Inport  Port=3
  Vx : Inport  Port=4
  Vy : Inport  Port=5
  Yaw rate : Inport  Port=6
  Delr : Inport  Port=7
  Add : Sum
  Add1 : Sum
  Add2 : Sum  Inputs=+-
  Divide : Product  Inputs=*/
  Product : Product  Inputs=3
  Product1 : Product  Inputs=3
  Trigonometric Function : Trigonometry
  Trigonometric Function1 : Trigonometry  Operator=cos
  Trigonometric Function2 : Trigonometry  Operator=atan
  alpfr : Outport
  wires:
  Add2/1 -> alpfr/1
  Delr/1 -> Add2/1
  Trigonometric Function2/1 -> Add2/2
  In2/1 -> Product/2
  Add1/1 -> Divide/2
  Trigonometric Function/1 -> Product/3
  Divide/1 -> Trigonometric Function2/1
  Product1/1 -> Add1/2
  Add/1 -> Divide/1
  Trigonometric Function1/1 -> Product1/3
  Rfcenter/1 -> Product1/2
  Product/1 -> Add/2
  Vx/1 -> Add1/1
  efr/1 -> Trigonometric Function/1, Trigonometric Function1/1
  Vy/1 -> Add/1
  Yaw rate/1 -> Product/1, Product1/1

== system vectoring2023/Side slip angle/alprl Subsystem ==
  Rrc : Inport
  In2 : Inport  Port=2
  erl : Inport  Port=3
  Vx : Inport  Port=4
  Vy : Inport  Port=5
  Yaw rate : Inport  Port=6
  Add : Sum  Inputs=+-
  Add1 : Sum  Inputs=+-
  Divide : Product  Inputs=*/
  Gain : Gain  Gain=-1
  Product : Product  Inputs=3
  Product1 : Product  Inputs=3
  Trigonometric Function : Trigonometry
  Trigonometric Function1 : Trigonometry  Operator=cos
  Trigonometric Function2 : Trigonometry  Operator=atan
  alprl : Outport
  wires:
  Gain/1 -> alprl/1
  Trigonometric Function2/1 -> Gain/1
  In2/1 -> Product/2
  Add1/1 -> Divide/2
  Trigonometric Function/1 -> Product/3
  Divide/1 -> Trigonometric Function2/1
  Product1/1 -> Add1/2
  Add/1 -> Divide/1
  Trigonometric Function1/1 -> Product1/3
  Rrc/1 -> Product1/2
  Product/1 -> Add/2
  Vx/1 -> Add1/1
  erl/1 -> Trigonometric Function/1, Trigonometric Function1/1
  Vy/1 -> Add/1
  Yaw rate/1 -> Product/1, Product1/1

== system vectoring2023/Side slip angle/alprr Subsystem1 ==
  Rrc : Inport
  In2 : Inport  Port=2
  err : Inport  Port=3
  Vx : Inport  Port=4
  Vy : Inport  Port=5
  Yaw rate : Inport  Port=6
  Add : Sum  Inputs=+-
  Add1 : Sum
  Divide : Product  Inputs=*/
  Gain : Gain  Gain=-1
  Product : Product  Inputs=3
  Product1 : Product  Inputs=3
  Trigonometric Function : Trigonometry  Operator=cos
  Trigonometric Function1 : Trigonometry
  Trigonometric Function2 : Trigonometry  Operator=atan
  alprr : Outport
  wires:
  Yaw rate/1 -> Product1/1, Product/1
  Vy/1 -> Add/1
  err/1 -> Trigonometric Function1/1, Trigonometric Function/1
  Vx/1 -> Add1/1
  Product/1 -> Add/2
  Rrc/1 -> Product1/2
  Trigonometric Function1/1 -> Product1/3
  Add/1 -> Divide/1
  Product1/1 -> Add1/2
  Divide/1 -> Trigonometric Function2/1
  Trigonometric Function/1 -> Product/3
  Add1/1 -> Divide/2
  In2/1 -> Product/2
  Trigonometric Function2/1 -> Gain/1
  Gain/1 -> alprr/1

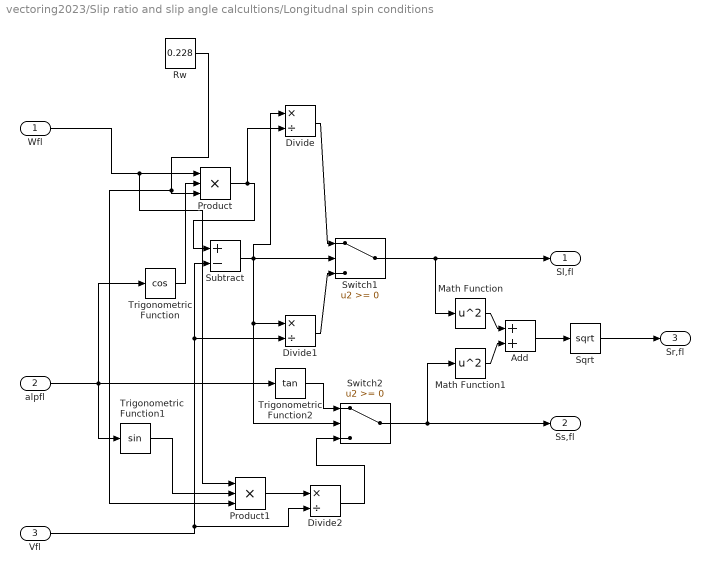
== system vectoring2023/Slip ratio and slip angle calcultions/Longitudnal spin conditions ==
  Wfl : Inport
  alpfl : Inport  Port=2
  Vfl : Inport  Port=3
  Add : Sum
  Divide : Product  Inputs=*/
  Divide1 : Product  Inputs=*/
  Divide2 : Product  Inputs=*/
  Math Function : Math  Operator=square
  Math Function1 : Math  Operator=square
  Product : Product  Inputs=3
  Product1 : Product  Inputs=3
  Rw : Constant  Value=0.228
  Sqrt : Sqrt
  Subtract : Sum  Inputs=+-
  Switch1 : Switch  SaturateOnIntegerOverflow=off  InputSameDT=off
  Switch2 : Switch  SaturateOnIntegerOverflow=off  InputSameDT=off
  Trigonometric Function : Trigonometry  Operator=cos
  Trigonometric Function1 : Trigonometry
  Trigonometric Function2 : Trigonometry  Operator=tan
  Sl,fl : Outport
  Ss,fl : Outport  Port=2
  Sr,fl : Outport  Port=3
  wires:
  Product/1 -> Divide/2, Subtract/1
  Divide/1 -> Switch1/1
  Wfl/1 -> Product1/1, Product/1
  Trigonometric Function/1 -> Product/2
  Subtract/1 -> Switch2/2, Divide1/1, Divide/1, Switch1/2
  alpfl/1 -> Trigonometric Function2/1, Trigonometric Function/1, Trigonometric Function1/1
  Rw/1 -> Product1/3, Product/3
  Divide1/1 -> Switch1/3
  Vfl/1 -> Divide2/2, Divide1/2, Subtract/2
  Switch1/1 -> Math Function/1, Sl,fl/1
  Trigonometric Function1/1 -> Product1/2
  Product1/1 -> Divide2/1
  Divide2/1 -> Switch2/3
  Switch2/1 -> Math Function1/1, Ss,fl/1
  Trigonometric Function2/1 -> Switch2/1
  Math Function/1 -> Add/1
  Math Function1/1 -> Add/2
  Add/1 -> Sqrt/1
  Sqrt/1 -> Sr,fl/1

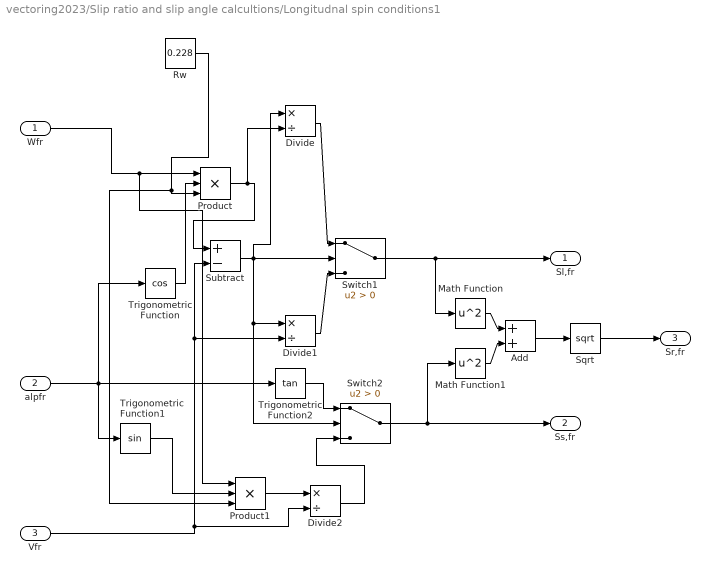
== system vectoring2023/Slip ratio and slip angle calcultions/Longitudnal spin conditions1 ==
  Wfr : Inport
  alpfr : Inport  Port=2
  Vfr : Inport  Port=3
  Add : Sum
  Divide : Product  Inputs=*/
  Divide1 : Product  Inputs=*/
  Divide2 : Product  Inputs=*/
  Math Function : Math  Operator=square
  Math Function1 : Math  Operator=square
  Product : Product  Inputs=3
  Product1 : Product  Inputs=3
  Rw : Constant  Value=0.228
  Sqrt : Sqrt
  Subtract : Sum  Inputs=+-
  Switch1 : Switch  Criteria=u2 > Threshold  SaturateOnIntegerOverflow=off  InputSameDT=off
  Switch2 : Switch  Criteria=u2 > Threshold  SaturateOnIntegerOverflow=off  InputSameDT=off
  Trigonometric Function : Trigonometry  Operator=cos
  Trigonometric Function1 : Trigonometry
  Trigonometric Function2 : Trigonometry  Operator=tan
  Sl,fr : Outport
  Ss,fr : Outport  Port=2
  Sr,fr : Outport  Port=3
  wires:
  Sqrt/1 -> Sr,fr/1
  Add/1 -> Sqrt/1
  Math Function1/1 -> Add/2
  Math Function/1 -> Add/1
  Trigonometric Function2/1 -> Switch2/1
  Switch2/1 -> Ss,fr/1, Math Function1/1
  Divide2/1 -> Switch2/3
  Product1/1 -> Divide2/1
  Trigonometric Function1/1 -> Product1/2
  Switch1/1 -> Sl,fr/1, Math Function/1
  Vfr/1 -> Subtract/2, Divide1/2, Divide2/2
  Divide1/1 -> Switch1/3
  Rw/1 -> Product/3, Product1/3
  alpfr/1 -> Trigonometric Function1/1, Trigonometric Function/1, Trigonometric Function2/1
  Subtract/1 -> Switch1/2, Divide/1, Divide1/1, Switch2/2
  Trigonometric Function/1 -> Product/2
  Wfr/1 -> Product/1, Product1/1
  Divide/1 -> Switch1/1
  Product/1 -> Subtract/1, Divide/2

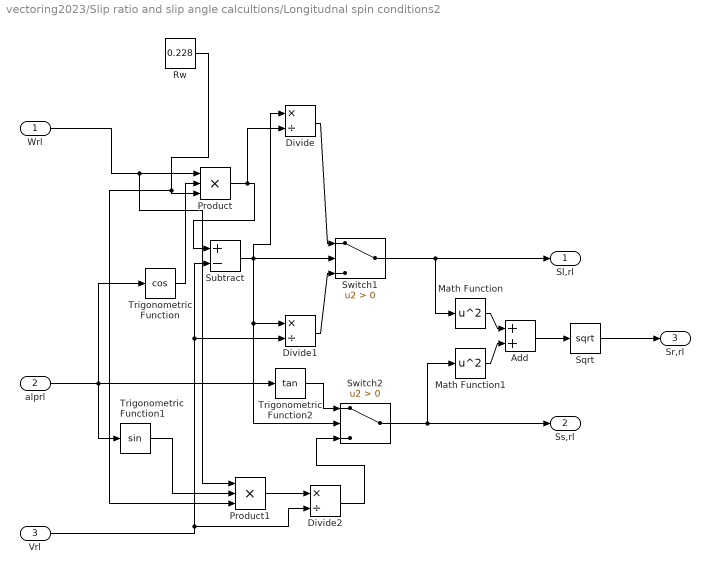
== system vectoring2023/Slip ratio and slip angle calcultions/Longitudnal spin conditions2 ==
  Wrl : Inport
  alprl : Inport  Port=2
  Vrl : Inport  Port=3
  Add : Sum
  Divide : Product  Inputs=*/
  Divide1 : Product  Inputs=*/
  Divide2 : Product  Inputs=*/
  Math Function : Math  Operator=square
  Math Function1 : Math  Operator=square
  Product : Product  Inputs=3
  Product1 : Product  Inputs=3
  Rw : Constant  Value=0.228
  Sqrt : Sqrt
  Subtract : Sum  Inputs=+-
  Switch1 : Switch  Criteria=u2 > Threshold  SaturateOnIntegerOverflow=off  InputSameDT=off
  Switch2 : Switch  Criteria=u2 > Threshold  SaturateOnIntegerOverflow=off  InputSameDT=off
  Trigonometric Function : Trigonometry  Operator=cos
  Trigonometric Function1 : Trigonometry
  Trigonometric Function2 : Trigonometry  Operator=tan
  Sl,rl : Outport
  Ss,rl : Outport  Port=2
  Sr,rl : Outport  Port=3
  wires:
  Product/1 -> Divide/2, Subtract/1
  Divide/1 -> Switch1/1
  Wrl/1 -> Product1/1, Product/1
  Trigonometric Function/1 -> Product/2
  Subtract/1 -> Switch2/2, Divide1/1, Divide/1, Switch1/2
  alprl/1 -> Trigonometric Function2/1, Trigonometric Function/1, Trigonometric Function1/1
  Rw/1 -> Product1/3, Product/3
  Divide1/1 -> Switch1/3
  Vrl/1 -> Divide2/2, Divide1/2, Subtract/2
  Switch1/1 -> Math Function/1, Sl,rl/1
  Trigonometric Function1/1 -> Product1/2
  Product1/1 -> Divide2/1
  Divide2/1 -> Switch2/3
  Switch2/1 -> Math Function1/1, Ss,rl/1
  Trigonometric Function2/1 -> Switch2/1
  Math Function/1 -> Add/1
  Math Function1/1 -> Add/2
  Add/1 -> Sqrt/1
  Sqrt/1 -> Sr,rl/1

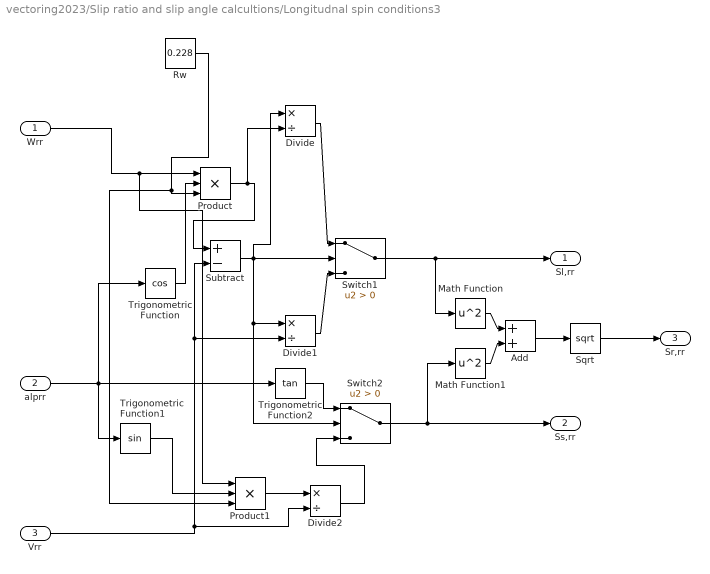
== system vectoring2023/Slip ratio and slip angle calcultions/Longitudnal spin conditions3 ==
  Wrr : Inport
  alprr : Inport  Port=2
  Vrr : Inport  Port=3
  Add : Sum
  Divide : Product  Inputs=*/
  Divide1 : Product  Inputs=*/
  Divide2 : Product  Inputs=*/
  Math Function : Math  Operator=square
  Math Function1 : Math  Operator=square
  Product : Product  Inputs=3
  Product1 : Product  Inputs=3
  Rw : Constant  Value=0.228
  Sqrt : Sqrt
  Subtract : Sum  Inputs=+-
  Switch1 : Switch  Criteria=u2 > Threshold  SaturateOnIntegerOverflow=off  InputSameDT=off
  Switch2 : Switch  Criteria=u2 > Threshold  SaturateOnIntegerOverflow=off  InputSameDT=off
  Trigonometric Function : Trigonometry  Operator=cos
  Trigonometric Function1 : Trigonometry
  Trigonometric Function2 : Trigonometry  Operator=tan
  Sl,rr : Outport
  Ss,rr : Outport  Port=2
  Sr,rr : Outport  Port=3
  wires:
  Sqrt/1 -> Sr,rr/1
  Add/1 -> Sqrt/1
  Math Function1/1 -> Add/2
  Math Function/1 -> Add/1
  Trigonometric Function2/1 -> Switch2/1
  Switch2/1 -> Ss,rr/1, Math Function1/1
  Divide2/1 -> Switch2/3
  Product1/1 -> Divide2/1
  Trigonometric Function1/1 -> Product1/2
  Switch1/1 -> Sl,rr/1, Math Function/1
  Vrr/1 -> Subtract/2, Divide1/2, Divide2/2
  Divide1/1 -> Switch1/3
  Rw/1 -> Product/3, Product1/3
  alprr/1 -> Trigonometric Function1/1, Trigonometric Function/1, Trigonometric Function2/1
  Subtract/1 -> Switch1/2, Divide/1, Divide1/1, Switch2/2
  Trigonometric Function/1 -> Product/2
  Wrr/1 -> Product/1, Product1/1
  Divide/1 -> Switch1/1
  Product/1 -> Subtract/1, Divide/2

== system vectoring2023/Slip ratio and slip angle calcultions/Wheel lateral X  ==
  In1 : Inport
  In2 : Inport  Port=2
  In3 : Inport  Port=3
  Add : Sum
  Product : Product
  Product1 : Product
  Trigonometric Function : Trigonometry
  Trigonometric Function1 : Trigonometry  Operator=cos
  Fwx,fl : Outport
  wires:
  Trigonometric Function1/1 -> Product/2
  Product/1 -> Add/1
  Add/1 -> Fwx,fl/1
  Trigonometric Function/1 -> Product1/1
  Product1/1 -> Add/2
  In3/1 -> Product1/2
  In2/1 -> Trigonometric Function/1, Trigonometric Function1/1
  In1/1 -> Product/1

== system vectoring2023/Slip ratio and slip angle calcultions/Wheel lateral X 1 ==
  Fwl : Inport
  alp : Inport  Port=2
  Fws : Inport  Port=3
  Add : Sum
  Product : Product
  Product1 : Product
  Trigonometric Function : Trigonometry
  Trigonometric Function1 : Trigonometry  Operator=cos
  Fwx,fr : Outport
  wires:
  Fwl/1 -> Product/1
  alp/1 -> Trigonometric Function1/1, Trigonometric Function/1
  Fws/1 -> Product1/2
  Product1/1 -> Add/2
  Trigonometric Function/1 -> Product1/1
  Add/1 -> Fwx,fr/1
  Product/1 -> Add/1
  Trigonometric Function1/1 -> Product/2

== system vectoring2023/Slip ratio and slip angle calcultions/Wheel lateral X 2 ==
  Fwl : Inport
  alp : Inport  Port=2
  Fws : Inport  Port=3
  Add : Sum
  Product : Product
  Product1 : Product
  Trigonometric Function : Trigonometry
  Trigonometric Function1 : Trigonometry  Operator=cos
  Fwx,rl : Outport
  wires:
  Trigonometric Function1/1 -> Product/2
  Product/1 -> Add/1
  Add/1 -> Fwx,rl/1
  Trigonometric Function/1 -> Product1/1
  Product1/1 -> Add/2
  Fws/1 -> Product1/2
  alp/1 -> Trigonometric Function/1, Trigonometric Function1/1
  Fwl/1 -> Product/1

== system vectoring2023/Slip ratio and slip angle calcultions/Wheel lateral X 3 ==
  Fwl : Inport
  alp : Inport  Port=2
  Fws : Inport  Port=3
  Add : Sum
  Product : Product
  Product1 : Product
  Trigonometric Function : Trigonometry
  Trigonometric Function1 : Trigonometry  Operator=cos
  Fwx,rr : Outport
  wires:
  Fwl/1 -> Product/1
  alp/1 -> Trigonometric Function1/1, Trigonometric Function/1
  Fws/1 -> Product1/2
  Product1/1 -> Add/2
  Trigonometric Function/1 -> Product1/1
  Add/1 -> Fwx,rr/1
  Product/1 -> Add/1
  Trigonometric Function1/1 -> Product/2

== system vectoring2023/Slip ratio and slip angle calcultions/Wheel longitudnal Y ==
  Fwl : Inport
  alp : Inport  Port=2
  Fws : Inport  Port=3
  Add : Sum  Inputs=-+
  Product : Product
  Product1 : Product
  Trigonometric Function : Trigonometry  Operator=cos
  Trigonometric Function1 : Trigonometry
  Fwy,fl : Outport
  wires:
  Fwl/1 -> Product/1
  alp/1 -> Trigonometric Function1/1, Trigonometric Function/1
  Fws/1 -> Product1/2
  Product1/1 -> Add/2
  Trigonometric Function/1 -> Product1/1
  Add/1 -> Fwy,fl/1
  Product/1 -> Add/1
  Trigonometric Function1/1 -> Product/2

== system vectoring2023/Slip ratio and slip angle calcultions/Wheel longitudnal Y1 ==
  Fwl : Inport
  alp : Inport  Port=2
  Fws : Inport  Port=3
  Add : Sum  Inputs=-+
  Product : Product
  Product1 : Product
  Trigonometric Function : Trigonometry  Operator=cos
  Trigonometric Function1 : Trigonometry
  Fwy,fr : Outport
  wires:
  Trigonometric Function1/1 -> Product/2
  Product/1 -> Add/1
  Add/1 -> Fwy,fr/1
  Trigonometric Function/1 -> Product1/1
  Product1/1 -> Add/2
  Fws/1 -> Product1/2
  alp/1 -> Trigonometric Function/1, Trigonometric Function1/1
  Fwl/1 -> Product/1

== system vectoring2023/Slip ratio and slip angle calcultions/Wheel longitudnal Y2 ==
  Fwl : Inport
  alp : Inport  Port=2
  Fws : Inport  Port=3
  Add : Sum  Inputs=-+
  Product : Product
  Product1 : Product
  Trigonometric Function : Trigonometry  Operator=cos
  Trigonometric Function1 : Trigonometry
  Fwy,rl : Outport
  wires:
  Fwl/1 -> Product/1
  alp/1 -> Trigonometric Function1/1, Trigonometric Function/1
  Fws/1 -> Product1/2
  Product1/1 -> Add/2
  Trigonometric Function/1 -> Product1/1
  Add/1 -> Fwy,rl/1
  Product/1 -> Add/1
  Trigonometric Function1/1 -> Product/2

== system vectoring2023/Slip ratio and slip angle calcultions/Wheel longitudnal Y3 ==
  Fwl : Inport
  alp : Inport  Port=2
  Fws : Inport  Port=3
  Add : Sum  Inputs=-+
  Product : Product
  Product1 : Product
  Trigonometric Function : Trigonometry  Operator=cos
  Trigonometric Function1 : Trigonometry
  Fwy,rr : Outport
  wires:
  Trigonometric Function1/1 -> Product/2
  Product/1 -> Add/1
  Add/1 -> Fwy,rr/1
  Trigonometric Function/1 -> Product1/1
  Product1/1 -> Add/2
  Fws/1 -> Product1/2
  alp/1 -> Trigonometric Function/1, Trigonometric Function1/1
  Fwl/1 -> Product/1

== system vectoring2023/Tire model/Subsystem1 ==
  Sl,fl : Inport
  Sr,fl : Inport  Port=2
  Ss,fl : Inport  Port=3
  Divide : Product  Inputs=*/
  Divide1 : Product  Inputs=*/
  Product : Product
  Product1 : Product
  Subsystem : Subsystem
  Ul,fl : Outport
  Us,fl : Outport  Port=2
  wires:
  Ss,fl/1 -> Divide1/1
  Subsystem/1(UrSfl) -> Product1/2, Product/2
  Product1/1 -> Us,fl/1
  Sl,fl/1 -> Divide/1
  Sr,fl/1 -> Divide1/2, Divide/2, Subsystem/1(In1)
  Product/1 -> Ul,fl/1
  Divide1/1 -> Product1/1
  Divide/1 -> Product/1

== system vectoring2023/Tire model/Subsystem2 ==
  Sl,fr : Inport
  Sr,fr : Inport  Port=2
  Ss,fr : Inport  Port=3
  Divide : Product  Inputs=*/
  Divide1 : Product  Inputs=*/
  Product : Product
  Product1 : Product
  Subsystem : Subsystem
  Ul,fr : Outport
  Us,fr : Outport  Port=2
  wires:
  Divide/1 -> Product/1
  Divide1/1 -> Product1/1
  Product/1 -> Ul,fr/1
  Sr,fr/1 -> Subsystem/1(In1), Divide/2, Divide1/2
  Sl,fr/1 -> Divide/1
  Product1/1 -> Us,fr/1
  Subsystem/1(UrSfl) -> Product/2, Product1/2
  Ss,fr/1 -> Divide1/1

== system vectoring2023/Tire model/Subsystem3 ==
  Sl,rl : Inport
  Sr,rl : Inport  Port=2
  Ss,rl : Inport  Port=3
  Divide : Product  Inputs=*/
  Divide1 : Product  Inputs=*/
  Product : Product
  Product1 : Product
  Subsystem : Subsystem
  Ul,rl : Outport
  Us,rl : Outport  Port=2
  wires:
  Ss,rl/1 -> Divide1/1
  Subsystem/1(UrSfl) -> Product1/2, Product/2
  Product1/1 -> Us,rl/1
  Sl,rl/1 -> Divide/1
  Sr,rl/1 -> Divide1/2, Divide/2, Subsystem/1(In1)
  Product/1 -> Ul,rl/1
  Divide1/1 -> Product1/1
  Divide/1 -> Product/1

== system vectoring2023/Tire model/Subsystem4 ==
  Sl,rr : Inport
  Sr,rr : Inport  Port=2
  Ss,rr : Inport  Port=3
  Divide : Product  Inputs=*/
  Divide1 : Product  Inputs=*/
  Product : Product
  Product1 : Product
  Subsystem : Subsystem
  Ul,rr : Outport
  Us,rr : Outport  Port=2
  wires:
  Divide/1 -> Product/1
  Divide1/1 -> Product1/1
  Product/1 -> Ul,rr/1
  Sr,rr/1 -> Subsystem/1(In1), Divide/2, Divide1/2
  Sl,rr/1 -> Divide/1
  Product1/1 -> Us,rr/1
  Subsystem/1(UrSfl) -> Product/2, Product1/2
  Ss,rr/1 -> Divide1/1

== system vectoring2023/Vertical load /Vertical Fores ==
  ax : Inport
  ay : Inport  Port=2
  Hcg : Constant  Value=0.813
  Vertical force fl : Subsystem
  Vertical force fr : Subsystem
  Vertical force rl : Subsystem
  Vertical force rr : Subsystem
  g : Constant  Value=9.81
  l : Constant  Value=1.29
  lf : Constant  Value=0.615
  lr : Constant  Value=0.665
  m : Constant  Value=356
  tf : Constant  Value=1.24
  tr : Constant  Value=1.24
  Fz,fl : Outport
  Fz,fr : Outport  Port=2
  Fz,rl : Outport  Port=3
  Fz,rr : Outport  Port=4
  wires:
  g/1 -> Vertical force rr/1(g), Vertical force rl/1(g), Vertical force fr/1(g), Vertical force fl/1(g)
  lf/1 -> Vertical force fr/2(lf), Vertical force fl/2(lf)
  l/1 -> Vertical force rr/3(l), Vertical force rl/3(l), Vertical force fr/3(l), Vertical force fl/3(l)
  ax/1 -> Vertical force fl/4(ax), Vertical force rr/4(ax), Vertical force rl/4(ax), Vertical force fr/4(ax)
  tf/1 -> Vertical force fr/6(tf), Vertical force fl/7(tf)
  ay/1 -> Vertical force rr/8(ay), Vertical force rl/8(ay), Vertical force fl/8(ay), Vertical force fr/7(ay)
  Vertical force fl/1(Fz,fl) -> Fz,fl/1
  m/1 -> Vertical force rr/5(m), Vertical force rl/5(m), Vertical force fr/5(m), Vertical force fl/5(m)
  Hcg/1 -> Vertical force fl/6(Hcg), Vertical force rr/6(Hcg), Vertical force rl/6(Hcg), Vertical force fr/8(Hcg)
  Vertical force fr/1(Fz,fr) -> Fz,fr/1
  lr/1 -> Vertical force rr/2(lr), Vertical force rl/2(lr)
  tr/1 -> Vertical force rr/7(tr), Vertical force rl/7(tr)
  Vertical force rl/1(Fz,rl) -> Fz,rl/1
  Vertical force rr/1(Fz,rr) -> Fz,rr/1

== system vectoring2023/Wheel Dynamics/Wfl subsystem ==
  Ffl : Inport
  -1/b : Gain  Gain=-1/0.1
  Discrete Derivative : simulink/Discrete/Discrete Derivative  gainval=1.0  ICPrevScaledInput=0.0  OutMin=[]  OutMax=[]  OutDataType=fixdt(1, 16)  OutScaling=2^-10  DoSatur=off
  Iw : Constant  Value=2.5
  Product : Product
  Product2 : Product
  Rw : Constant  Value=0.228
  Sum : Sum  Inputs=|++
  Unit Delay : UnitDelay  SampleTime=-1  HasFrameUpgradeWarning=on
  Wfl : Outport
  wires:
  Sum/1 -> -1/b/1
  Iw/1 -> Product2/1
  Product2/1 -> Sum/2
  Discrete Derivative/1 -> Product2/2
  Ffl/1 -> Product/2
  -1/b/1 -> Unit Delay/1, Wfl/1
  Product/1 -> Sum/1
  Rw/1 -> Product/1
  Unit Delay/1 -> Discrete Derivative/1

== system vectoring2023/Wheel Dynamics/Wfr subsytem ==
  Ffr : Inport
  -1/b1 : Gain  Gain=-1/0.1
  Discrete Derivative : simulink/Discrete/Discrete Derivative  gainval=1.0  ICPrevScaledInput=0.0  OutMin=[]  OutMax=[]  OutDataType=fixdt(1, 16)  OutScaling=2^-10  DoSatur=off
  Iw1 : Constant  Value=2.5
  Product1 : Product
  Product3 : Product
  Rw1 : Constant  Value=0.228
  Sum1 : Sum  Inputs=|++
  Unit Delay : UnitDelay  SampleTime=-1  HasFrameUpgradeWarning=on
  Wfr : Outport
  wires:
  Product1/1 -> Sum1/1
  Product3/1 -> Sum1/2
  Rw1/1 -> Product1/1
  -1/b1/1 -> Unit Delay/1, Wfr/1
  Iw1/1 -> Product3/1
  Ffr/1 -> Product1/2
  Discrete Derivative/1 -> Product3/2
  Sum1/1 -> -1/b1/1
  Unit Delay/1 -> Discrete Derivative/1
